simulink model "S32K344_LED"  (R2023b)
settings: Solver=FixedStepAuto  StartTime=0.0  StopTime=10.0  RelTol=1e-3
PreLoadFcn:
  | % NXP_MBDT_S32K3 callback: DO NOT REMOVE
  | mbd_s32k3.common.nxp.model_callbacks.preLoadFcn();
PostLoadFcn:
  | % NXP_MBDT_S32K3 callback: DO NOT REMOVE
  | mbd_s32k3.common.nxp.model_callbacks.postLoadFcn();
InitFcn:
  | % NXP_MBDT_S32K3 callback: DO NOT REMOVE
  | mbd_s32k3.common.nxp.model_callbacks.initFcn();
libraries: simulink x2, mbd_s32k3_io_library x2, mbd_s32k3_utility_library x1, mbd_s32k3_cdd_library x1
settings Model: DataDictionary=S32K344_LED.sldd  Creator=HUAWEI  LastModifiedBy=HUAWEI
settings OptimizationCC: EnhancedBackFolding=on  PassReuseOutputArgsAs=Individual arguments  ZeroExternalMemoryAtStartup=off  ZeroInternalMemoryAtStartup=off  MaxStackSize=64  OptimizeBlockOrder=speed  DifferentSizesBufferReuse=on  OptimizationCustomize=off  EfficientTunableParamExpr=on
settings DebuggingCC: ParameterTunabilityLossMsg=error
settings HardwareCC: ProdBitPerPointer=32  ProdBitPerSizeT=32  ProdBitPerPtrDiffT=32  ProdLargestAtomicInteger=Long  ProdLargestAtomicFloat=Double  ProdWordSize=32  ProdHWDeviceType=ARM Compatible->ARM Cortex
settings SFSimCC: MATLABDynamicMemAlloc=off
settings RTWCC: Description=Embedded Coder  SystemTargetFile=ert.tlc  HardwareBoard=NXP S32K3xx  TemplateMakefile=ert_default_tmf  Toolchain=S32DS GCC  BuildConfiguration=Faster Runs
settings CodeAppCC: ForceParamTrailComments=on  IgnoreCustomStorageClasses=off  OperatorAnnotations=on  SimulinkDataObjDesc=on  SFDataObjDesc=on  InsertBlockDesc=on
settings ERTTargetCC: ExtModeTransport=1  ExtModeMexFile=ext_serial_win32_comm  ERTSrcFileBannerTemplate=mbd_s32k3_ert_code_template.cgt  ERTHdrFileBannerTemplate=mbd_s32k3_ert_code_template.cgt  ERTDataSrcFileTemplate=mbd_s32k3_ert_code_template.cgt  ERTDataHdrFileTemplate=mbd_s32k3_ert_code_template.cgt

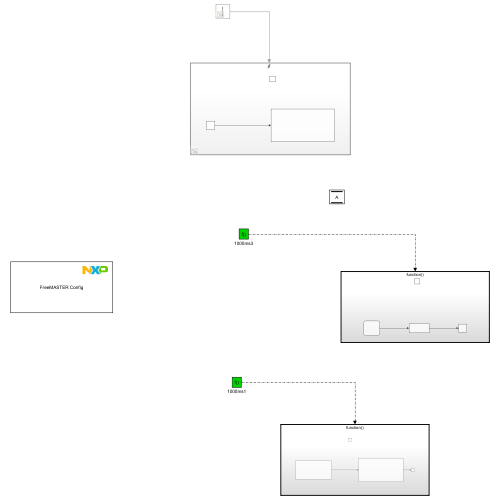
[thumbnail: Simulink's stored preview of the top-level diagram]
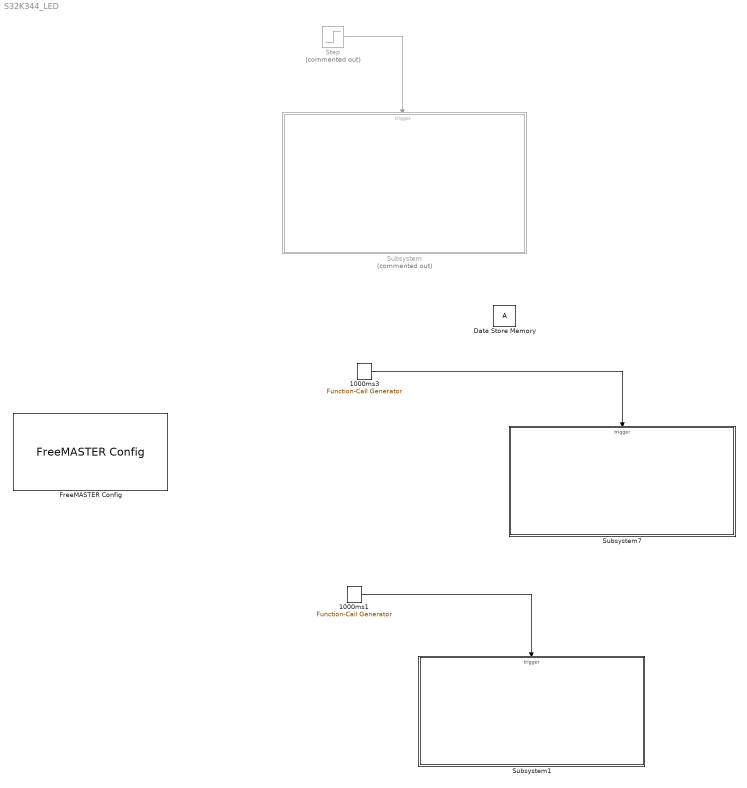
== system S32K344_LED ==
  1000ms1 : simulink/Ports & Subsystems/Function-Call Generator  Priority=4  sample_time=1  numberOfIterations=1  DisallowWideOutput=off
  1000ms3 : simulink/Ports & Subsystems/Function-Call Generator  Priority=4  sample_time=1  numberOfIterations=1  DisallowWideOutput=off
  Data Store Memory : DataStoreMemory  WriteAfterWriteMsg=warning  ShowAdditionalParam=off  OutDataTypeStr=uint8
  FreeMASTER Config : mbd_s32k3_utility_library/FreeMASTER blocks/FreeMASTER Config  connection_type=Serial  instance=LPUART_6  baudrate=115200  isr_prio=5  mode=Short Interrupt  scope_use=1  scope_max_vars=8  automatic_buff_size=on  buff_size=255  default_rfifo_size=on  rfifo_size=32
  Step : Step  Commented=on
  Subsystem : Subsystem  Commented=on
  Subsystem1 : Subsystem
  Subsystem7 : Subsystem
  wires:
  Step/1 -> Subsystem/Trigger
  1000ms3/1 -> Subsystem7/Trigger
  1000ms1/1 -> Subsystem1/Trigger

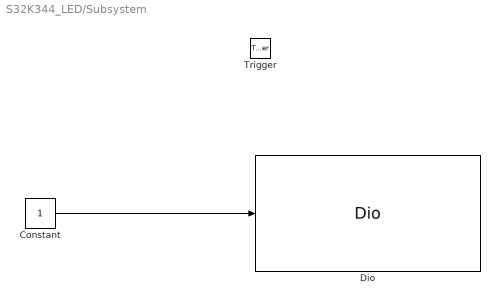
== system S32K344_LED/Subsystem ==
  Trigger : TriggerPort  VariantControl=(inherit)
  Constant : Constant  OutDataTypeStr=uint8
  Dio : mbd_s32k3_io_library/Dio  api_func=Dio_WriteChannel  channel=RGBLED0_BLUE  channel_group=No channel groups configured  port=No ports configured  gpioSim=on  text=<binary blob, 2198 chars, not shown>
  wires:
  Constant/1 -> Dio/1

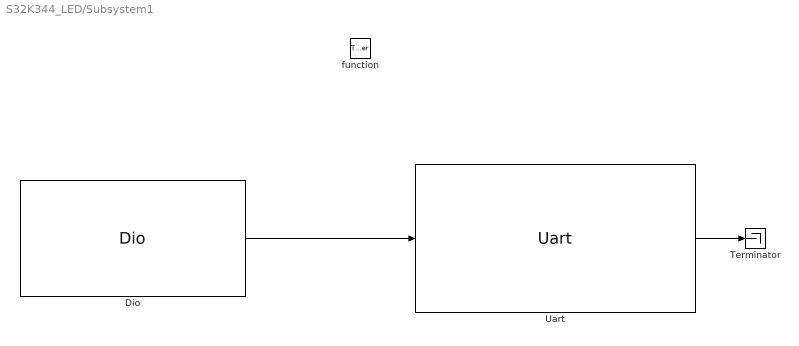
== system S32K344_LED/Subsystem1 ==
  function : TriggerPort  TriggerType=function-call  VariantControl=Variant
  Dio : mbd_s32k3_io_library/Dio  api_func=Dio_ReadChannel  channel=RGBLED0_BLUE  channel_group=No channel groups configured  port=No ports configured  gpioSim=off  text=<binary blob, 2198 chars, not shown>
  Terminator : Terminator
  Uart : mbd_s32k3_cdd_library/Uart  api_func=Uart_SyncSend  channel=UartChannel_0  baudrate=UART_BAUDRATE_1200  transfer_type=UART_SEND  timeout=0  text=<binary blob, 2472 chars, not shown>
  wires:
  Uart/1 -> Terminator/1
  Dio/1 -> Uart/1

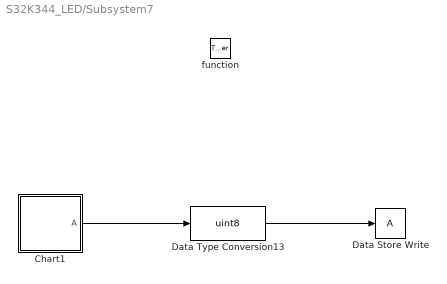
== system S32K344_LED/Subsystem7 ==
  function : TriggerPort  TriggerType=function-call  VariantControl=Variant
  Chart1 : Stateflow chart  TreatAsAtomicUnit=on
  Data Store Write : DataStoreWrite  IndexOptions=Index vector (dialog)  Indices=1  OutputSizes=1
  Data Type Conversion13 : DataTypeConversion  OutDataTypeStr=uint8  SaturateOnIntegerOverflow=off  RndMeth=Floor
  wires:
  Chart1/1(" A") -> Data Type Conversion13/1
  Data Type Conversion13/1 -> Data Store Write/1

== stateflow chart S32K344_LED/Subsystem7/Chart1 ==
  state A
  state A1
  (default) -> A
  A -> A1
  A1 -> A
  data: A output boolean [0..1]
